simulink model "practice8_2"  (Simulink 7.9)
settings: Solver=ode45  StartTime=0.0  StopTime=15  RelTol=1e-3
settings Model: Creator=sony  LastModifiedBy=sony

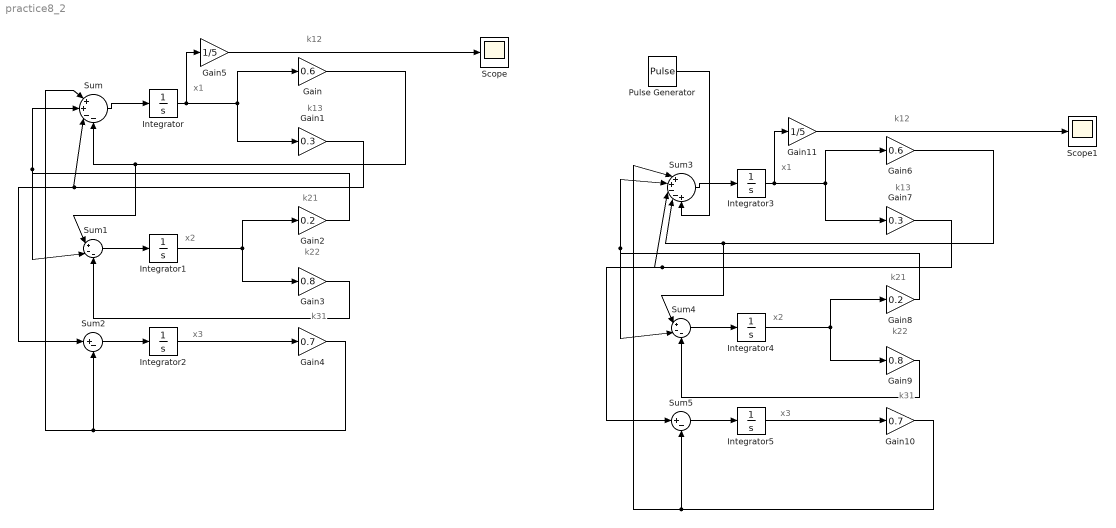
== system practice8_2 ==
  note: k12
  note: k13
  note: k21
  note: k22
  note: k31
  note: x1
  note: x2
  note: x3
  note: k12
  note: k13
  note: k21
  note: k22
  note: k31
  note: x1
  note: x2
  note: x3
  Gain : Gain  Gain=0.6
  Gain1 : Gain  Gain=0.3
  Gain10 : Gain  Gain=0.7
  Gain11 : Gain  Gain=1/5
  Gain2 : Gain  Gain=0.2
  Gain3 : Gain  Gain=0.8
  Gain4 : Gain  Gain=0.7
  Gain5 : Gain  Gain=1/5
  Gain6 : Gain  Gain=0.6
  Gain7 : Gain  Gain=0.3
  Gain8 : Gain  Gain=0.2
  Gain9 : Gain  Gain=0.8
  Integrator : Integrator  InitialCondition=200
  Integrator{1..2,4..5} (4 alike) : Integrator
  Integrator3 : Integrator  InitialCondition=400
  Pulse Generator : DiscretePulseGenerator  PulseType=Time based  Amplitude=200/0.02
  Scope : Scope
  Scope1 : Scope
  Sum : Sum  Inputs=|++--
  Sum1 : Sum  Inputs=|+--
  Sum2 : Sum  Inputs=|+-
  Sum3 : Sum  Inputs=|++--+
  Sum4 : Sum  Inputs=|+--
  Sum5 : Sum  Inputs=|+-
  wires:
  Sum/1 -> Integrator/1
  Integrator/1 -> Gain/1, Gain1/1, Gain5/1
  Integrator1/1 -> Gain2/1, Gain3/1
  Integrator2/1 -> Gain4/1
  Gain2/1 -> Sum1/2, Sum/2
  Gain4/1 -> Sum2/2, Sum/1
  Gain1/1 -> Sum2/1, Sum/3
  Gain/1 -> Sum1/1, Sum/4
  Sum1/1 -> Integrator1/1
  Gain3/1 -> Sum1/3
  Sum2/1 -> Integrator2/1
  Gain5/1 -> Scope/1
  Sum3/1 -> Integrator3/1
  Integrator3/1 -> Gain6/1, Gain7/1, Gain11/1
  Integrator4/1 -> Gain8/1, Gain9/1
  Integrator5/1 -> Gain10/1
  Gain8/1 -> Sum4/2, Sum3/2
  Gain10/1 -> Sum5/2, Sum3/1
  Gain7/1 -> Sum5/1, Sum3/3
  Gain6/1 -> Sum4/1, Sum3/4
  Sum4/1 -> Integrator4/1
  Gain9/1 -> Sum4/3
  Sum5/1 -> Integrator5/1
  Gain11/1 -> Scope1/1
  Pulse Generator/1 -> Sum3/5
